simulink library "CTRL_LO_ST1"  (R2023b)
settings: Solver=VariableStepAuto  StartTime=0.0  StopTime=10.0  RelTol=1e-3
libraries: CTRL_LO_ST1_DFLATLGT x1, CTRL_LO_ST1_LGTFDIS x1, CTRL_LO_ST1_WHFSUM x1, CTRL_LO_ST1_YAWTRQLAT x1, CTRL_LO_ST1_YAWTRQLATDIST x1, CTRL_LO_ST1_YAWTRQLGT x1, CTRL_LO_ST1_YAWTRQLGTDIST x1, CTRL_LO_ST1_YAWTRQSUM x1, CTRL_LO_ST1_TRQDMDWHL x1
settings Model: Creator=blatak  LastModifiedBy=blatak

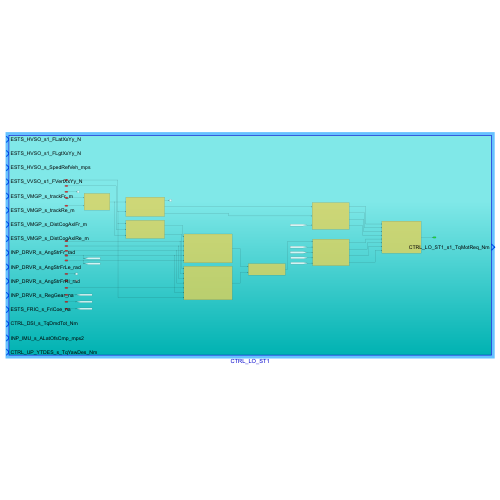
[thumbnail: Simulink's stored preview of the top-level diagram]
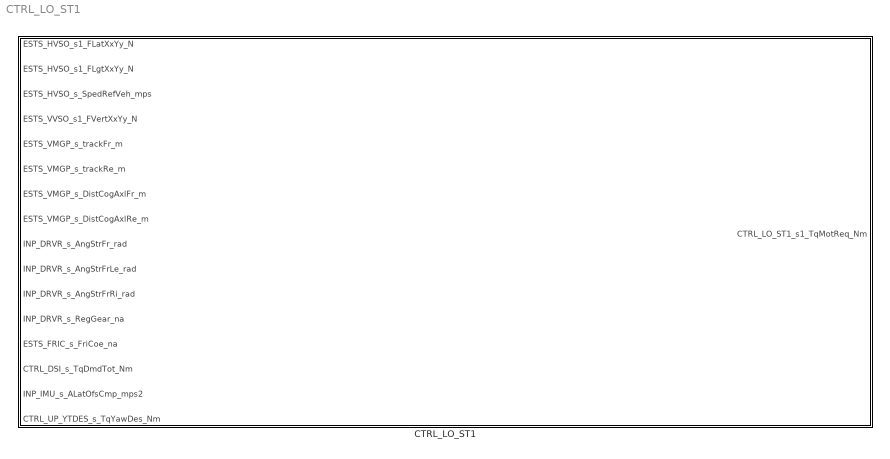
== system CTRL_LO_ST1 ==
  CTRL_LO_ST1 : Subsystem

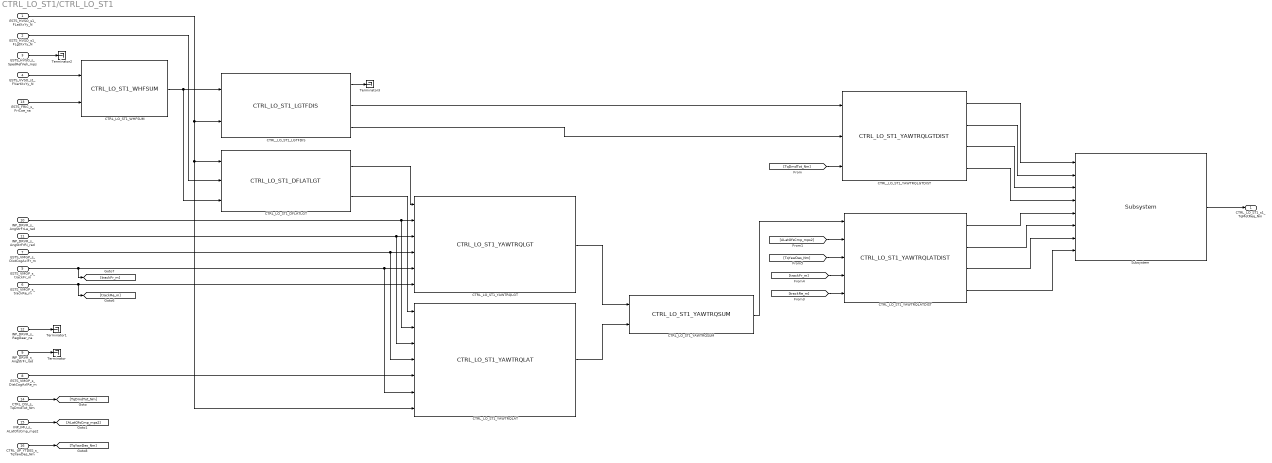
== system CTRL_LO_ST1/CTRL_LO_ST1 ==
  ESTS_HVSO_s1_FLatXxYy_N : Inport
  ESTS_HVSO_s1_FLgtXxYy_N : Inport  Port=2
  ESTS_HVSO_s_SpedRefVeh_mps : Inport  Port=3
  ESTS_VVSO_s1_FVertXxYy_N : Inport  Port=4
  ESTS_VMGP_s_trackFr_m : Inport  Port=5
  ESTS_VMGP_s_trackRe_m : Inport  Port=6
  ESTS_VMGP_s_DistCogAxlFr_m : Inport  Port=7
  ESTS_VMGP_s_DistCogAxlRe_m : Inport  Port=8
  INP_DRVR_s_AngStrFr_rad : Inport  Port=9
  INP_DRVR_s_AngStrFrLe_rad : Inport  Port=10
  INP_DRVR_s_AngStrFrRi_rad : Inport  Port=11
  INP_DRVR_s_RegGear_na : Inport  Port=12
  ESTS_FRIC_s_FriCoe_na : Inport  Port=13
  CTRL_DSI_s_TqDmdTot_Nm : Inport  Port=14
  INP_IMU_s_ALatOfsCmp_mps2 : Inport  Port=15
  CTRL_UP_YTDES_s_TqYawDes_Nm : Inport  Port=16
  CTRL_LO_ST1_DFLATLGT : CTRL_LO_ST1_DFLATLGT/CTRL_LO_ST1_DFLATLGT  SystemSampleTime=-1  VariantActivationTime=update diagram  AllowFlexibleInterface=on  Latency=0  AutoFrameSizeCalculation=off
  CTRL_LO_ST1_LGTFDIS : CTRL_LO_ST1_LGTFDIS/CTRL_LO_ST1_LGTFDIS  SystemSampleTime=-1  VariantActivationTime=update diagram  AllowFlexibleInterface=on  Latency=0  AutoFrameSizeCalculation=off
  CTRL_LO_ST1_WHFSUM : CTRL_LO_ST1_WHFSUM/CTRL_LO_ST1_WHFSUM  SystemSampleTime=-1  VariantActivationTime=update diagram  AllowFlexibleInterface=on  Latency=0  AutoFrameSizeCalculation=off
  CTRL_LO_ST1_YAWTRQLAT : CTRL_LO_ST1_YAWTRQLAT/CTRL_LO_ST1_YAWTRQLAT  SystemSampleTime=-1  VariantActivationTime=update diagram  AllowFlexibleInterface=on  Latency=0  AutoFrameSizeCalculation=off
  CTRL_LO_ST1_YAWTRQLATDIST : CTRL_LO_ST1_YAWTRQLATDIST/CTRL_LO_ST1_YAWTRQLATDIST  SystemSampleTime=-1  VariantActivationTime=update diagram  AllowFlexibleInterface=on  Latency=0  AutoFrameSizeCalculation=off
  CTRL_LO_ST1_YAWTRQLGT : CTRL_LO_ST1_YAWTRQLGT/CTRL_LO_ST1_YAWTRQLGT  SystemSampleTime=-1  VariantActivationTime=update diagram  AllowFlexibleInterface=on  Latency=0  AutoFrameSizeCalculation=off
  CTRL_LO_ST1_YAWTRQLGTDIST : CTRL_LO_ST1_YAWTRQLGTDIST/CTRL_LO_ST1_YAWTRQLGTDIST  SystemSampleTime=-1  VariantActivationTime=update diagram  AllowFlexibleInterface=on  Latency=0  AutoFrameSizeCalculation=off
  CTRL_LO_ST1_YAWTRQSUM : CTRL_LO_ST1_YAWTRQSUM/CTRL_LO_ST1_YAWTRQSUM  SystemSampleTime=-1  VariantActivationTime=update diagram  AllowFlexibleInterface=on  Latency=0  AutoFrameSizeCalculation=off
  Subsystem : CTRL_LO_ST1_TRQDMDWHL/Subsystem  SystemSampleTime=-1  VariantActivationTime=update diagram  AllowFlexibleInterface=on  Latency=0  AutoFrameSizeCalculation=off
  Terminator{,1..3} (4 alike) : Terminator
  CTRL_LO_ST1_s1_TqMotReq_Nm : Outport
  wires:
  ESTS_VVSO_s1_FVertXxYy_N/1 -> CTRL_LO_ST1_WHFSUM/1
  ESTS_FRIC_s_FriCoe_na/1 -> CTRL_LO_ST1_WHFSUM/2
  CTRL_LO_ST1_WHFSUM/1 -> CTRL_LO_ST1_DFLATLGT/3, CTRL_LO_ST1_LGTFDIS/1
  ESTS_HVSO_s1_FLatXxYy_N/1 -> CTRL_LO_ST1_YAWTRQLAT/7, CTRL_LO_ST1_DFLATLGT/1, CTRL_LO_ST1_LGTFDIS/2
  ESTS_HVSO_s1_FLgtXxYy_N/1 -> CTRL_LO_ST1_DFLATLGT/2
  CTRL_LO_ST1_DFLATLGT/1 -> CTRL_LO_ST1_YAWTRQLGT/1
  INP_DRVR_s_AngStrFrLe_rad/1 -> CTRL_LO_ST1_YAWTRQLAT/2, CTRL_LO_ST1_YAWTRQLGT/2
  INP_DRVR_s_AngStrFrRi_rad/1 -> CTRL_LO_ST1_YAWTRQLAT/3, CTRL_LO_ST1_YAWTRQLGT/3
  ESTS_VMGP_s_DistCogAxlFr_m/1 -> CTRL_LO_ST1_YAWTRQLAT/4, CTRL_LO_ST1_YAWTRQLGT/4
  ESTS_VMGP_s_trackFr_m/1 -> [trackFr_m], CTRL_LO_ST1_YAWTRQLAT/6, CTRL_LO_ST1_YAWTRQLGT/5
  ESTS_VMGP_s_trackRe_m/1 -> [trackRe_m], CTRL_LO_ST1_YAWTRQLGT/6
  ESTS_VMGP_s_DistCogAxlRe_m/1 -> CTRL_LO_ST1_YAWTRQLAT/5
  CTRL_LO_ST1_DFLATLGT/2 -> CTRL_LO_ST1_YAWTRQLAT/1
  INP_DRVR_s_AngStrFr_rad/1 -> Terminator/1
  INP_DRVR_s_RegGear_na/1 -> Terminator1/1
  CTRL_LO_ST1_YAWTRQLGT/1 -> CTRL_LO_ST1_YAWTRQSUM/1
  CTRL_LO_ST1_YAWTRQLAT/1 -> CTRL_LO_ST1_YAWTRQSUM/2
  ESTS_HVSO_s_SpedRefVeh_mps/1 -> Terminator2/1
  CTRL_DSI_s_TqDmdTot_Nm/1 -> [TqDmdTot_Nm]
  CTRL_LO_ST1_LGTFDIS/2 -> CTRL_LO_ST1_YAWTRQLGTDIST/1
  CTRL_LO_ST1_LGTFDIS/3 -> CTRL_LO_ST1_YAWTRQLGTDIST/2
  [TqDmdTot_Nm] -> CTRL_LO_ST1_YAWTRQLGTDIST/3
  CTRL_LO_ST1_LGTFDIS/1 -> Terminator3/1
  INP_IMU_s_ALatOfsCmp_mps2/1 -> [ALatOfsCmp_mps2]
  CTRL_LO_ST1_YAWTRQSUM/1 -> CTRL_LO_ST1_YAWTRQLATDIST/1
  [ALatOfsCmp_mps2] -> CTRL_LO_ST1_YAWTRQLATDIST/2
  [trackFr_m] -> CTRL_LO_ST1_YAWTRQLATDIST/4
  [trackRe_m] -> CTRL_LO_ST1_YAWTRQLATDIST/5
  CTRL_UP_YTDES_s_TqYawDes_Nm/1 -> [TqYawDes_Nm]
  [TqYawDes_Nm] -> CTRL_LO_ST1_YAWTRQLATDIST/3
  Subsystem/1 -> CTRL_LO_ST1_s1_TqMotReq_Nm/1
  CTRL_LO_ST1_YAWTRQLGTDIST/1 -> Subsystem/1
  CTRL_LO_ST1_YAWTRQLGTDIST/2 -> Subsystem/2
  CTRL_LO_ST1_YAWTRQLGTDIST/3 -> Subsystem/3
  CTRL_LO_ST1_YAWTRQLGTDIST/4 -> Subsystem/4
  CTRL_LO_ST1_YAWTRQLATDIST/1 -> Subsystem/5
  CTRL_LO_ST1_YAWTRQLATDIST/2 -> Subsystem/6
  CTRL_LO_ST1_YAWTRQLATDIST/3 -> Subsystem/7
  CTRL_LO_ST1_YAWTRQLATDIST/4 -> Subsystem/8
